simulink model "test_for_Lk"  (R2015a)
settings: Solver=ode45  StartTime=0.0  StopTime=10.0  RelTol=1e-3
values from neighbouring files (symbols this model uses):
  A = [0 -87.2734439167 0 0 0 0 87.2734439167 -1.74546887833 0 0 0 0 ... (36 elements, 6x6)]    [A.mat]    (also in A_decompose.m = 0.01*[-0.773996386153021,96.9795539479971,0,0,0,0;-96.400970)
  B = [0  0; 43537  27917; 0  0; 192690  -42273; 0  0; -338240  439030]    [B.mat]    (also in B_decompose.m = 0.01*[-0.230745598618469,-0.153904745996477;0.06127775595526)
  C = [0 -5.1012 0 4.026 0 3.2726]    [C.mat]    (also in C_decompose.m = 0.01*[-23.1554338545303,9.56281796834669,0.435674513053965,-)
  H = [0 -5.4265 0 5.0795 0 5.0035]    [H.mat]
  Lk = [-59.477792404 31.7484157566 3951.54702126 -4057.82953256 6373.12577438 -2161.86440143]    [Lk.mat]
libraries: simulink x2
settings Model: Creator=p4wp4w  LastModifiedBy=p4wp4w

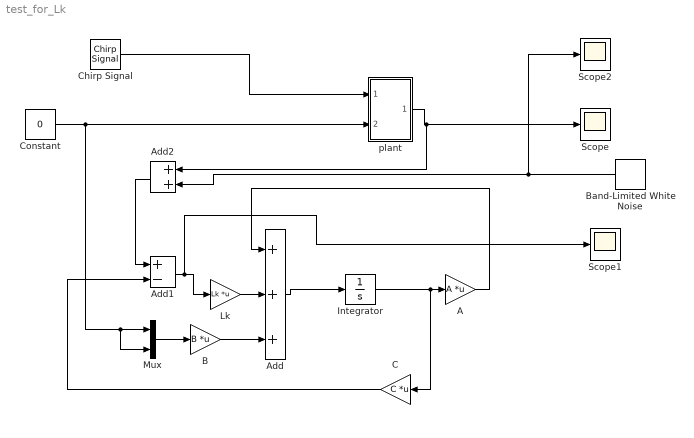
== system test_for_Lk ==
  A : Gain  Gain=A  Multiplication=Matrix(K*u)
  Add : Sum  Inputs=+++
  Add1 : Sum  Inputs=+-
  Add2 : Sum
  B : Gain  Gain=B  Multiplication=Matrix(K*u)
  Band-Limited White Noise : simulink/Sources/Band-Limited White Noise  Cov=[0.000001]  Ts=0.001  seed=[23341]
  C : Gain  Gain=C  Multiplication=Matrix(K*u)
  Chirp Signal : simulink/Sources/Chirp Signal  f1=0.1  T=10  f2=100
  Constant : Constant  Value=0
  Integrator : Integrator
  Lk : Gain  Gain=Lk  Multiplication=Matrix(K*u)
  Mux : Mux  Inputs=2
  Scope : Scope
  Scope1 : Scope
  Scope2 : Scope
      settings: SaveName=ScopeData2
  plant : Subsystem
  wires:
  Chirp Signal/1 -> plant/1(In1)
  Add/1 -> Integrator/1
  A/1 -> Add/1
  Integrator/1 -> C/1, A/1
  Mux/1 -> B/1
  Constant/1 -> Mux/2, Mux/1, plant/2(In2)
  plant/1(Out1) -> Add2/1, Scope/1
  C/1 -> Add1/2
  Lk/1 -> Add/2
  Add1/1 -> Scope1/1, Lk/1
  B/1 -> Add/3
  Add2/1 -> Add1/1
  Band-Limited White Noise/1 -> Scope2/1, Add2/2

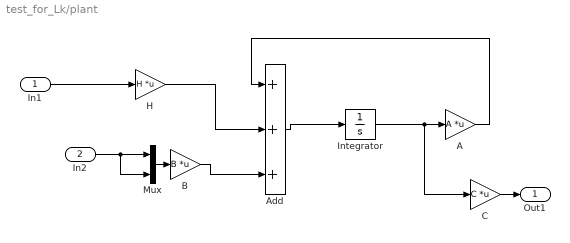
== system test_for_Lk/plant ==
  In1 : Inport
  In2 : Inport  Port=2
  A : Gain  Gain=A  Multiplication=Matrix(K*u)
  Add : Sum  Inputs=+++
  "B " : Gain  Gain=B  Multiplication=Matrix(K*u)
  C : Gain  Gain=C  Multiplication=Matrix(K*u)
  H : Gain  Gain=H  Multiplication=Matrix(K*u)
  Integrator : Integrator
  Mux : Mux  Inputs=2
  Out1 : Outport
  wires:
  Add/1 -> Integrator/1
  In1/1 -> H/1
  A/1 -> Add/1
  H/1 -> Add/2
  C/1 -> Out1/1
  Integrator/1 -> C/1, A/1
  Mux/1 -> "B "/1
  In2/1 -> Mux/2, Mux/1
  "B "/1 -> Add/3
